simulink model "SOGI"  (R2022b)
settings: Solver=VariableStepAuto  StartTime=0.0  StopTime=1  MaxStep=1e-7  RelTol=1e-5
undefined symbols (not defined in the file): DiscIntNeverNeededParam
settings Model: Creator=SSC  LastModifiedBy=SSC

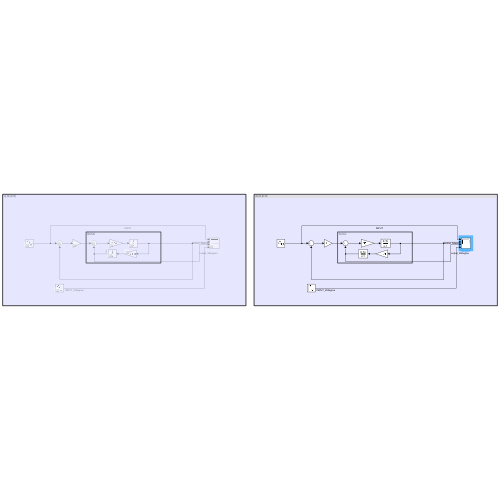
[thumbnail: Simulink's stored preview of the top-level diagram]
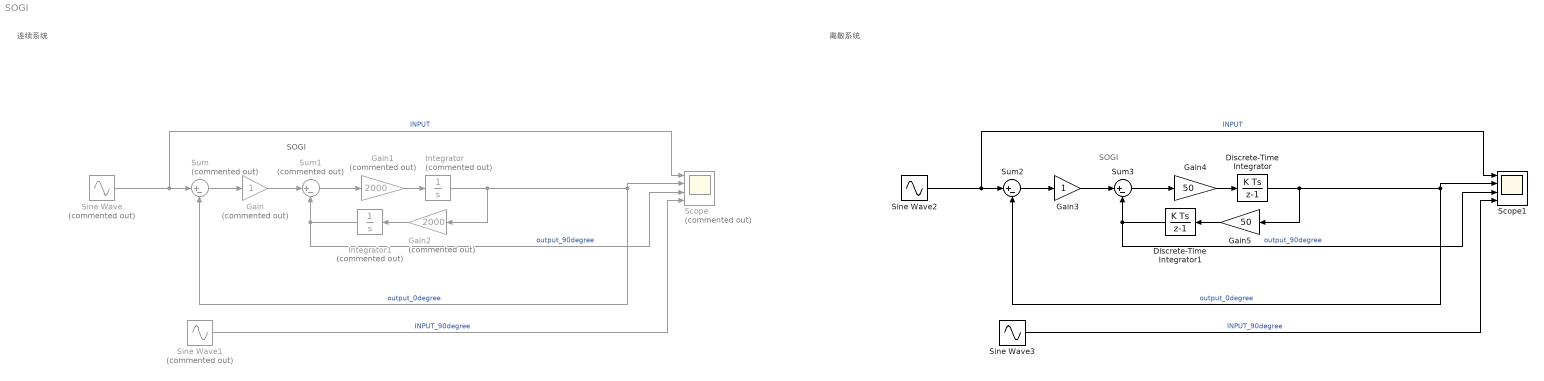
== system SOGI ==
  note: 连续系统
  note: SOGI
  note: 离散系统
  note: SOGI
  Discrete-Time Integrator : DiscreteIntegrator  SampleTime=1e-4  ICPrevOutput=DiscIntNeverNeededParam  ICPrevScaledInput=DiscIntNeverNeededParam
  Discrete-Time Integrator1 : DiscreteIntegrator  SampleTime=1e-4  ICPrevOutput=DiscIntNeverNeededParam  ICPrevScaledInput=DiscIntNeverNeededParam
  Gain : Gain  Commented=on
  Gain1 : Gain  Commented=on  Gain=2000
  Gain2 : Gain  Commented=on  Gain=2000
  Gain3 : Gain
  Gain4 : Gain  Gain=50
  Gain5 : Gain  Gain=50
  Integrator : Integrator  Commented=on
  Integrator1 : Integrator  Commented=on
  Scope : Scope  Commented=on  NumInputPorts=4
  Scope1 : Scope  NumInputPorts=4
  Sine Wave : Sin  Commented=on  Frequency=2000  SampleTime=0
  Sine Wave1 : Sin  Commented=on  Frequency=2000  Phase=-pi/2  SampleTime=0
  Sine Wave2 : Sin  Frequency=50  SampleTime=1e-4
  Sine Wave3 : Sin  Frequency=50  Phase=-pi/2  SampleTime=1e-4
  Sum : Sum  Commented=on  Inputs=|+-
  Sum1 : Sum  Commented=on  Inputs=|+-
  Sum2 : Sum  Inputs=|+-
  Sum3 : Sum  Inputs=|+-
  wires:
  Sum/1 -> Gain/1
  Sine Wave/1 -> Scope/1, Sum/1  "INPUT"
  Gain/1 -> Sum1/1
  Sum1/1 -> Gain1/1
  Gain1/1 -> Integrator/1
  Gain2/1 -> Integrator1/1
  Integrator/1 -> Gain2/1, Sum/2, Scope/2  "output_0degree"
  Integrator1/1 -> Sum1/2, Scope/3  "output_90degree"
  Sine Wave1/1 -> Scope/4  "INPUT_90degree"
  Sine Wave3/1 -> Scope1/4  "INPUT_90degree"
  Discrete-Time Integrator/1 -> Gain5/1, Sum2/2, Scope1/2  "output_0degree"
  Discrete-Time Integrator1/1 -> Sum3/2, Scope1/3  "output_90degree"
  Sum2/1 -> Gain3/1
  Gain3/1 -> Sum3/1
  Gain4/1 -> Discrete-Time Integrator/1
  Sum3/1 -> Gain4/1
  Sine Wave2/1 -> Scope1/1, Sum2/1  "INPUT"
  Gain5/1 -> Discrete-Time Integrator1/1
